simulink model "trabalho"  (R2024b)
settings: Solver=FixedStepAuto  StartTime=0.0  StopTime=15  FixedStep=0.001  RelTol=1e-3
settings DebuggingCC: AlgebraicLoopMsg=none

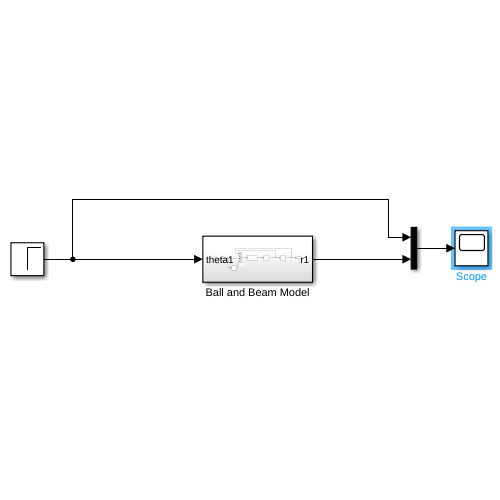
[thumbnail: Simulink's stored preview of the top-level diagram]
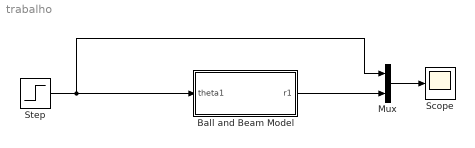
== system trabalho ==
  Ball and Beam Model : Subsystem
  Mux : Mux  Inputs=2
  Scope : Scope
  Step : Step  Time=0  After=0.15  SampleTime=0
  wires:
  Mux/1 -> Scope/1
  Ball and Beam Model/1(r1) -> Mux/2
  Step/1 -> Ball and Beam Model/1(theta1), Mux/1

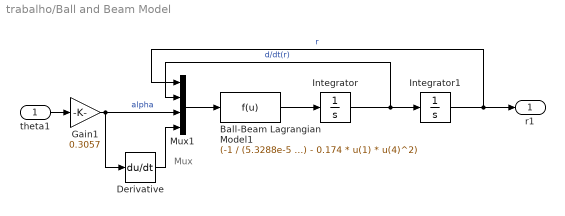
== system trabalho/Ball and Beam Model ==
  note: Mux
  theta1 : Inport
  Ball-Beam Lagrangian Model1 : Fcn  Expr=(-1 / (5.3288e-5 / (0.0175^2) + 0.174)) * (0.174 * (-9.8) * sin(u(3)) - 0.174 * u(1) * u(4)^2)
  Derivative : Derivative
  Gain1 : Gain  Gain=0.3057
  Integrator : Integrator
  Integrator1 : Integrator
  Mux1 : Mux
  r1 : Outport
  wires:
  Integrator1/1 -> Mux1/1, r1/1  "r"
  Mux1/1 -> Ball-Beam Lagrangian Model1/1
  theta1/1 -> Gain1/1
  Derivative/1 -> Mux1/4
  Gain1/1 -> Derivative/1, Mux1/3  "alpha"
  Integrator/1 -> Mux1/2, Integrator1/1  "d/dt(r)"
  Ball-Beam Lagrangian Model1/1 -> Integrator/1
